simulink model "ARFWr_Sim"  (R2025a)
settings: Solver=ode4  StartTime=0.0  StopTime=simLapStop  FixedStep=2e-4  RelTol=1e-3
PreLoadFcn:
  | % T2.3 ROLLING-START SEAM.
  | %
  | % Plant.slx's model workspace owns plantVx0 (T2.2 report section 4: "a seam,
  | % not a defect"), which drives BOTH the body's xbdot_o and all four tyre blocks'
  | % omegao -- so a rolling start can never be issued with stationary wheels.
  | % Its stored default is 0. This callback pushes the ACTIVE speed target at the
  | % start line into it, so the rolling start matches whatever drvVScale /
  | % drvUsePlan the driver is running with. Plant.slx is NOT this task's file, so
  | % it is not edited: the value is pushed into the loaded model workspace and
  | % Plant's dirty flag is restored, leaving the .slx on disk untouched.
  | %
  | % The vehicle's start POSE needs no push at all -- the reference path in
  | % DriverPath's model workspace was rigidly transformed at build time so that its
  | % first point is the origin with heading 0, which is exactly Plant's stored
  | % Xe_o = eul_o = [0 0 0].
  | %
  | % WHY PreLoadFcn AND NOT InitFcn: a referenced model's workspace is READ-ONLY
  | % once simulation starts. Doing this from InitFcn fails with
  | % Simulink:Libraries:WSLockViolation, "Attempt to modify a read-only model
  | % workspace" -- measured in T2.3. PreLoadFcn runs at load time, outside the lock.
  | %
  | % CONSEQUENCE, and the one thing to know before changing the speed target by
  | % hand: this fires ONCE, when ARFWr_Sim is loaded. If you edit drvVScale or
  | % drvUsePlan in DriverPath's model workspace afterwards and press Run, plantVx0
  | % is STALE and the car starts at the previous speed. Re-run this callback:
  | %     eval(get_param('ARFWr_Sim','PreLoadFcn'))
  | % Scripted runs should instead override it on the SimulationInput, which is
  | % immune to the ordering:
  | %     si = si.setVariable('plantVx0', v0, 'Workspace', 'Plant')
  | load_system('DriverPath');
  | load_system('Plant');
  | mwD = get_param('DriverPath','ModelWorkspace');
  | if mwD.getVariable('drvUsePlan') > 0.5
  |     vProf = mwD.getVariable('drvRefVplan');
  | else
  |     vProf = mwD.getVariable('drvRefVraw');
  | end
  | v0 = mwD.getVariable('drvVScale')*vProf(1);
  | mwP = get_param('Plant','ModelWorkspace');
  | dirty0 = get_param('Plant','Dirty');
  | if ~isequal(mwP.getVariable('plantVx0'), v0)
  |     mwP.assignin('plantVx0', v0);
  |     set_param('Plant','Dirty', dirty0);
  | end
InitFcn:
  | % LIVE INSTRUMENTS -- the DISPLAY-ONLY indicated-gear rule.
  | % indicatedGearParams is the SINGLE owner of ratios/omPk/omCap/nHold, shared
  | % with simulink/viz/indicatedGear.m (the burned-in HUD digit), so the live
  | % Dashboard digit and the recorded video digit cannot drift apart. The plant
  | % runs ONE fixed ratio and never shifts -- see that function's header.
  | hudGear = indicatedGearParams(pt);
model workspace (MAT data in the model file):
  simLapStop = 183
undefined symbols (not defined in the file): Sim3dSensor, vp
libraries: sim3dlib x5, sim3dautolib x1
Description:
  | ARFWr_Sim -- top closed-loop harness (T2.3). NEVER code-generated.
  | 
  | DriverPath -> Plant -> Sensors -> AeroECU -> Plant (wings + TV).
  | Rates: Plant 1 kHz ode4, AeroECU 100 Hz discrete (ecuTs), driver continuous on
  | the parent's 1 ms step.
  | 
  | VARIANTS (both LABEL mode, so the active choice is stored in this .slx and no
  | base-workspace variant control variables are needed):
  |   Scenario Source {ClosedLoop | Replay}  -- ClosedLoop active.
  |   Visualization   {Off | Dashboard | Unreal3D} -- Off active.
  | 
  | SIMULATION PACING is ON at 1x in the saved model, which is what a demo run
  | wants. Every measurement run in T2.3 was made UNPACED, by overriding
  | EnablePacing on a Simulink.SimulationInput -- pacing would make a wall-clock
  | ratio measurement meaningless.
  | 
  | ROLLING START: see this model's InitFcn callback.
  | 
  | STATUS OF THE MODELLING LAYERS (was "PLACEHOLDERS STILL LIVE" until T4.2):
  |   tyres  LIVE  -- per-axle Pacejka MF5.2 (T3.2), gate 1 passes at round-off.
  |   aero   LIVE  -- instantaneous ride-height map + both wing layers (T3.4),
  |                   gate 2 passes; the plant block matches aeroLiveEval to 1e-12.
  |   ECU    LIVE  -- reactive dual-wing law (gate 5, 96/97 % law fidelity) plus,
  |                   since T4.2, the front-axle TV allocator on SensorBus.kappaRef
  |                   and .TqAxle. tv.enable in simulink/params/tvParams.m switches
  |                   TV off at build time.
  |   driver APPROXIMATE -- a forward-time Stanley + traction-pedal-map driver, NOT
  |                   an optimal-control solution. It completes a clean BCN lap in
  |                   138.3 s against the offline solve's 102.674 s (gate 6,
  |                   simulink/validation/validateClosedLoop.m, which prints the
  |                   full wing-schedule and grip-utilisation evidence). Quote the
  |                   gate's own numbers, never an extrapolated partial lap.
settings Model: DataDictionary=ARFWr_RT.sldd  Creator=ASUS  LastModifiedBy=ASUS
settings DataIOCC: SignalLoggingName=simLog
settings DebuggingCC: AlgebraicLoopMsg=error  UnconnectedInputMsg=error  UnconnectedOutputMsg=error  UnconnectedLineMsg=error

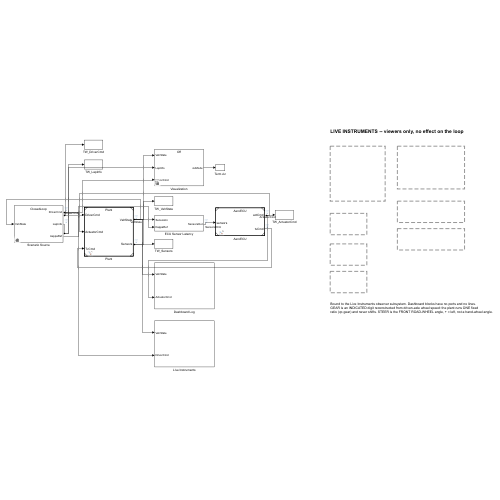
[thumbnail: Simulink's stored preview of the top-level diagram]
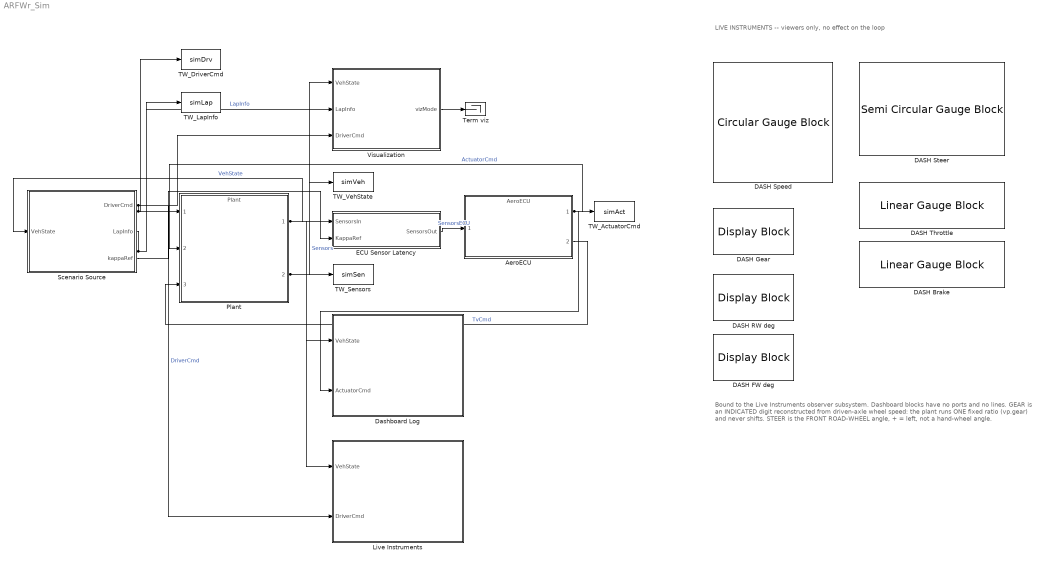
== system ARFWr_Sim ==
  note: LIVE INSTRUMENTS -- viewers only, no effect on the loop
  note: Bound to the Live Instruments observer subsystem. Dashboard blocks have no ports and no lines.
      | GEAR is an INDICATED digit reconstructed from driven-axle wheel speed: the plant runs ONE fixed
      | ratio (vp.gear) and never shifts. STEER is the FRONT ROAD-WHEEL angle, + = left, not a hand-wheel angle.
  AeroECU : ModelReference  Description=AeroECU (T1.1-T1.5), 100 Hz discrete (ecuTs = 0.01). Sensors in, ActuatorCmdBus + TvCmdBus out. NOT tuned or touched by T2.3.  ModelNameDialog=AeroECU  SimulationMode=Normal  ModelReferenceVersion=1.7
  DASH Brake : LinearGaugeBlock  Description="BRAKE  %"  LabelPosition=Bottom  FontColor=[0.0, 0.0, 0.0]
  DASH FW deg : DisplayBlock  Description="FRONT FLAP alphaFW_pos  [deg]"  LabelPosition=Bottom  Transparency=1  GridColor=[0.502, 0.502, 0.502]
  DASH Gear : DisplayBlock  Description=GEAR (indicated) -- plant runs one ratio, never shifts  LabelPosition=Bottom  Transparency=1  GridColor=[0.502, 0.502, 0.502]
  DASH RW deg : DisplayBlock  Description="REAR WING alphaRW_pos  [deg]"  LabelPosition=Bottom  Transparency=1  GridColor=[0.502, 0.502, 0.502]
  DASH Speed : CircularGaugeBlock  Description="SPEED  km/h"  LabelPosition=Bottom  ScaleMax=360  FontColor=[0.0, 0.0, 0.0]
  DASH Steer : SemiCircularGaugeBlock  Description="STEER road-wheel, + = left  [deg]"  LabelPosition=Bottom  ScaleMin=-15  ScaleMax=15  FontColor=[0.0, 0.0, 0.0]
  DASH Throttle : LinearGaugeBlock  Description="THROTTLE  %"  LabelPosition=Bottom  FontColor=[0.0, 0.0, 0.0]
  Dashboard Log : Subsystem  Description=|
      | T5.2 dashboard logging tap (simulink/viz/dashboardApp.m's SIGNAL-NAME CONTRACT).
      | Pure observer: two Inports branch the existing VehState and ActuatorCmd lines,
      | nothing is fed back into the loop and every output ends in a Terminator, so the
      | closed loop is bit-identical with this subsystem present or deleted.
      | 
      | Every logged port uses DataLoggingNameMode = Custom, so the logsout element name
      | is fixed by this block and cannot drift with a line label:
      |   vehState.x vehState.y           -- flat elements whose NAME carries the dot
      |   vx                              -- plant truth off VehStateBus (NOT the
      |                                      latency-delayed SensorBus copy)
      | alphaRW_pos / alphaFW_pos are NOT tapped here: Plant.slx already logs both
      | under exactly those names, and two same-named Dataset elements break
      | getElement(name) lookup (it returns a Dataset of the matches, not an
      | element). The tap copy was measured bit-identical to Plant's.
      |   stationRW stationFW sOn         -- ActuatorCmdBus; the stations are the
      |                                      1-BASED INDEX the contract asks for, not degrees
      |   aeroClF aeroClR aeroCd          -- optional north-star downforce/drag panel
  ECU Sensor Latency : Subsystem  Description=|
      | ONE-SAMPLE (1 ms) SENSOR LATENCY on the Plant -> AeroECU path. This is the
      | ALGEBRAIC-LOOP BREAK for the ECU half of the closed loop -- the driver half is
      | broken separately, inside DriverPath (see its Sensor delay block).
      | 
      | MEASURED, not assumed. Wiring Plant.Sensors straight into AeroECU.sensors gives:
      |   Simulink:Engine:BlockWithStatesModifiedInOutputUpdateInAlgLoop
      |     "ARFWr_Sim/Plant or the model referenced by it contains a block that updates
      |      persistent or state variables while computing outputs and is not supported
      |      in an algebraic loop"
      |   Simulink:Engine:BlkWithPortInLoop  input ports (1,2,3,4) of ARFWr_Sim/AeroECU
      |   Simulink:Engine:BlkWithPortInLoop  input ports (4..9) of ARFWr_Sim/Plant
      | i.e. Sensors -> ECU -> ActuatorCmd/TvCmd -> Plant -> Sensors. The offending
      | stateful block is the VDB Combined Slip Wheel 2DOF (its Wheel Module clutch
      | updates state while computing outputs), which is the same block T2.2 already had
      | to break with a Memory on the Omega feedback -- see Plant/Omega Memory.
      | 
      | PHYSICALLY HONEST, not a workaround: the ECU is a 100 Hz sampled controller
      | reading sensors over a bus. One 1 ms sample of acquisition latency is an order
      | of magnitude LESS than the 10 ms the controller already waits between its own
      | steps, so it changes nothing the ECU can observe.
      | 
      | Mux/Demux around the Memory because SensorBus is a VIRTUAL bus and Memory does
      | not accept one. Channel order is the Bus Selector's: vx, r, Tbrake, TbMax.
  Live Instruments : Subsystem  Description=|
      | LIVE INSTRUMENTS -- pure observer for the root Dashboard blocks.
      | 
      | Two Inports BRANCH the existing top-level VehState (Plant/1) and DriverCmd
      | (Scenario Source/1) lines. Nothing is fed back into the loop and every signal
      | ends in a Terminator, so the closed loop is bit-identical with this subsystem
      | present or deleted -- the same contract as the Dashboard Log tap next door.
      | 
      | Display units, so the gauges read what a driver would read:
      |   Speed kmh    = vx * 3.6            [km/h]
      |   Steer deg    = steer * 180/pi      [deg, FRONT ROAD-WHEEL angle, + = LEFT --
      |                                       NOT a hand-wheel angle; peak ~11 deg]
      |   Throttle pct = accel * 100         [%, POST traction ceiling]
      |   Brake pct    = brake * 100         [%, POST traction ceiling]
      |   alphaRW_pos / alphaFW_pos pass through unscaled -- already degrees.
      | 
      | GEAR OBSERVER -- DISPLAY ONLY, and the caveat travels with the number.
      | Plant.slx models ONE fixed effective ratio (vp.gear) and NEVER SHIFTS; the
      | supplier 8-speed table pt.gearbox is read by nothing in the plant or the
      | solver. This block reconstructs a legibility digit from driven-axle wheel
      | speed at 0.05 s, the same rule and the same parameters as
      | simulink/viz/indicatedGear.m (single owner: indicatedGearParams). No shift
      | event, torque interruption, ratio step or inertia change exists anywhere in
      | the simulation, and no reported result depends on this digit. It must never
      | appear in a lap-time, shift-strategy or powertrain statement.
      | 
      | Every gear parameter arrives as a Constant whose Value is a hudGear field, so
      | there is no numeric literal in the gear path. hudGear is built by the model
      | InitFcn as indicatedGearParams(pt).
  Plant : ModelReference  Description=|  ModelNameDialog=Plant  SimulationMode=Normal  ModelReferenceVersion=1.14
      | Plant.slx (T2.2), 1 kHz ode4. In: DriverCmd, ActuatorCmd, TvCmd. Out: VehState
      | (full state, ISO 8855), Sensors (the four channels the ECU consumes).
      | Not touched by T2.3 -- see this model's InitFcn for the one runtime value
      | (plantVx0) that is pushed into its model workspace and immediately un-dirtied.
  Scenario Source : Subsystem  Description=|  Variant=on  VariantControlMode=label  LabelModeActiveChoice=ClosedLoop
      | ScenarioSource variant (design spec decision 2, "closed loop + replay mode").
      | Label mode; active choice ClosedLoop. Both choices take VehStateBus in and
      | produce DriverCmdBus + a 12-element LapInfo vector out.
  TW_ActuatorCmd : ToWorkspace  VariableName=simAct  SaveFormat=Structure With Time  SampleTime=-1
  TW_DriverCmd : ToWorkspace  VariableName=simDrv  SaveFormat=Structure With Time  SampleTime=-1
  TW_LapInfo : ToWorkspace  VariableName=simLap  SaveFormat=Structure With Time  SampleTime=-1
  TW_Sensors : ToWorkspace  VariableName=simSen  SaveFormat=Structure With Time  SampleTime=-1
  TW_VehState : ToWorkspace  VariableName=simVeh  SaveFormat=Structure With Time  SampleTime=-1
  Term viz : Terminator
  Visualization : Subsystem  Description=|  Variant=on  VariantControlMode=label  LabelModeActiveChoice=Off
      | Visualization variant (design spec decision 10: "Viz outside RT boundary").
      | Label mode; active choice Off. All three choices take VehState + LapInfo and
      | return a scalar vizMode indicator (0 Off, 1 Dashboard, 2 Unreal3D) so the
      | active choice is observable in a log without opening the model.
      | 
      | All three choices are implemented: Off is a pure pass-through terminator
      | (T5.0), Dashboard is the logged-lap replay dashboard (T5.1/T5.2), Unreal3D
      | is the live sim3d scene (T5.3). None is a stub.
  wires:
  ECU Sensor Latency/1(SensorsOut) -> AeroECU/1  "SensorsECU"
  Scenario Source/1(DriverCmd) -> Plant/1, TW_DriverCmd/1, Live Instruments/2(DriverCmd), Visualization/3(DriverCmd)  "DriverCmd"
  Scenario Source/2(LapInfo) -> Visualization/2(LapInfo), TW_LapInfo/1  "LapInfo"
  Plant/1 -> Scenario Source/1(VehState), Visualization/1(VehState), TW_VehState/1, Dashboard Log/1(VehState), Live Instruments/1(VehState)  "VehState"
  AeroECU/1 -> Plant/2, TW_ActuatorCmd/1, Dashboard Log/2(ActuatorCmd)  "ActuatorCmd"
  Plant/2 -> TW_Sensors/1, ECU Sensor Latency/1(SensorsIn)  "Sensors"
  AeroECU/2 -> Plant/3  "TvCmd"
  Visualization/1(vizMode) -> Term viz/1
  Scenario Source/3(kappaRef) -> ECU Sensor Latency/2(KappaRef)

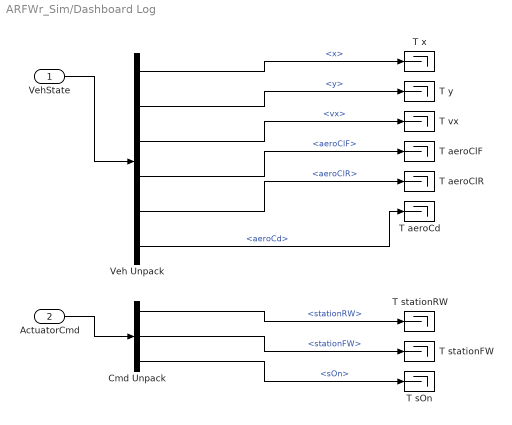
== system ARFWr_Sim/Dashboard Log ==
  VehState : Inport
  ActuatorCmd : Inport  Port=2
  Cmd Unpack : BusSelector  OutputSignals=stationRW,stationFW,sOn
  T aeroCd : Terminator
  T aeroClF : Terminator
  T aeroClR : Terminator
  T sOn : Terminator
  T stationFW : Terminator
  T stationRW : Terminator
  T vx : Terminator
  T x : Terminator
  T y : Terminator
  Veh Unpack : BusSelector  OutputSignals=x,y,vx,aeroClF,aeroClR,aeroCd
  wires:
  VehState/1 -> Veh Unpack/1
  ActuatorCmd/1 -> Cmd Unpack/1
  Veh Unpack/1 -> T x/1  "<x>"
  Veh Unpack/2 -> T y/1  "<y>"
  Veh Unpack/3 -> T vx/1  "<vx>"
  Veh Unpack/4 -> T aeroClF/1  "<aeroClF>"
  Veh Unpack/5 -> T aeroClR/1  "<aeroClR>"
  Veh Unpack/6 -> T aeroCd/1  "<aeroCd>"
  Cmd Unpack/1 -> T stationRW/1  "<stationRW>"
  Cmd Unpack/2 -> T stationFW/1  "<stationFW>"
  Cmd Unpack/3 -> T sOn/1  "<sOn>"

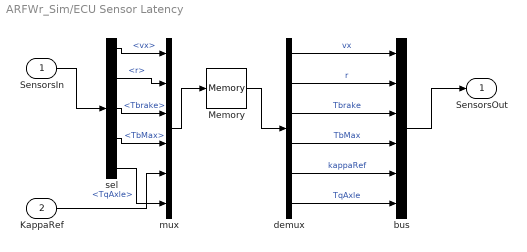
== system ARFWr_Sim/ECU Sensor Latency ==
  SensorsIn : Inport  OutDataTypeStr=Bus: SensorBus
  KappaRef : Inport  Description=Path curvature at the preview point, ISO [1/m], straight from the Scenario Source. It is muxed in as SensorBus element 5 INSTEAD of the element the Plant publishes (which is a hard 0 -- the plant has no path knowledge). Delayed by the same one 1 ms Memory sample as the plant channels so the ECU sees one consistent sensor snapshot.  Port=2
  Memory : Memory  Description=|  InitialCondition=[0; 0; 0; vp.Tbrake_max; 0; 0]
      | Initial condition [0; 0; 0; vp.Tbrake_max].
      | 
      | The fourth entry MUST be vp.Tbrake_max and MUST NOT be left at 0. SensorBus.TbMax
      | is the POSITIVE brake-torque magnitude cap, and the reactive law's brake trigger
      | (Functions/rwVelocityTarget.m's brakeSwitch, ported into AeroECU) uses an onset
      | width of w1frac*TbMax -- so a zero TbMax on the very first step divides by zero
      | inside the tanh argument. This is the same contract Plant's Vehicle State Bus
      | subsystem documents ("TbMax > 0 ALWAYS").
      | 
      | vx = r = Tbrake = 0 for one 1 ms step is harmless: kap2 = r^2/(vx^2+1) is 0
      | there, and Tbrake = 0 simply means "not braking" on step one.
  bus : BusCreator  Inputs=6  OutDataTypeStr=Bus: SensorBus
  demux : Demux  Outputs=6
  mux : Mux  Inputs=6
  sel : BusSelector  OutputSignals=vx,r,Tbrake,TbMax,TqAxle
  SensorsOut : Outport  OutDataTypeStr=Bus: SensorBus
  wires:
  SensorsIn/1 -> sel/1
  sel/1 -> mux/1  "<vx>"
  demux/1 -> bus/1  "vx"
  sel/2 -> mux/2  "<r>"
  demux/2 -> bus/2  "r"
  sel/3 -> mux/3  "<Tbrake>"
  demux/3 -> bus/3  "Tbrake"
  sel/4 -> mux/4  "<TbMax>"
  demux/4 -> bus/4  "TbMax"
  mux/1 -> Memory/1
  Memory/1 -> demux/1
  bus/1 -> SensorsOut/1
  sel/5 -> mux/6  "<TqAxle>"
  KappaRef/1 -> mux/5
  demux/5 -> bus/5  "kappaRef"
  demux/6 -> bus/6  "TqAxle"

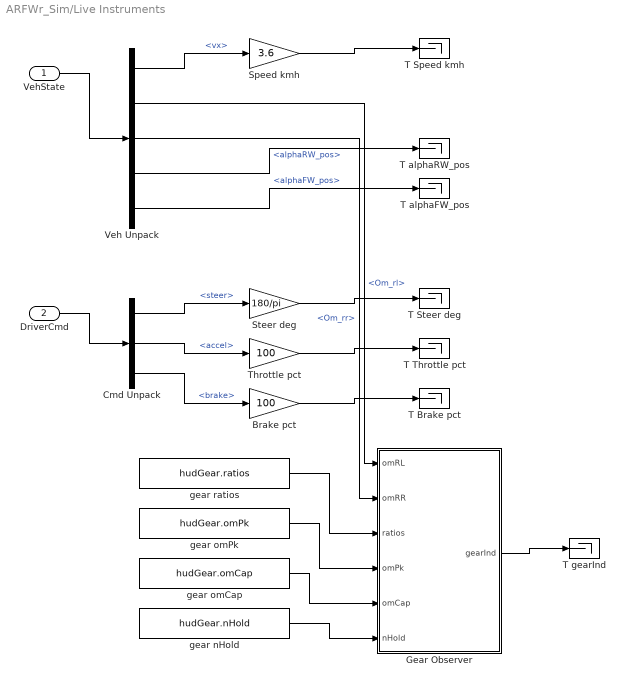
== system ARFWr_Sim/Live Instruments ==
  VehState : Inport
  DriverCmd : Inport  Port=2
  Brake pct : Gain  Description=DriverCmdBus.brake [0..1, POST traction ceiling] -> percent. Sampled at 0.05 s; display only.  Gain=100  SampleTime=0.05
  Cmd Unpack : BusSelector  OutputSignals=steer,accel,brake
  Gear Observer : MATLAB Function  Description=|  TreatAsAtomicUnit=on
      | DISPLAY-ONLY indicated gear, live. Reproduces simulink/viz/indicatedGear.m's
      | rule sample by sample: of the eight candidate crank speeds omWheel*ratios,
      | take the one nearest omPk among those at or under omCap (all over cap -> top
      | gear), then hold the digit until a new candidate has persisted nHold samples.
      | The plant runs ONE fixed ratio and never shifts -- this digit is a legibility
      | aid, never a shift model, and no reported result depends on it.
  Speed kmh : Gain  Description=vx [m/s] -> km/h for the speed Gauge. Sampled at 0.05 s; display only.  Gain=3.6  SampleTime=0.05
  Steer deg : Gain  Description=DriverCmdBus.steer [rad] -> deg. FRONT ROAD-WHEEL angle, + = LEFT, NOT a hand-wheel angle. Sampled at 0.05 s; display only.  Gain=180/pi  SampleTime=0.05
  T Brake pct : Terminator
  T Speed kmh : Terminator
  T Steer deg : Terminator
  T Throttle pct : Terminator
  T alphaFW_pos : Terminator
  T alphaRW_pos : Terminator
  T gearInd : Terminator
  Throttle pct : Gain  Description=DriverCmdBus.accel [0..1, POST traction ceiling] -> percent. Sampled at 0.05 s; display only.  Gain=100  SampleTime=0.05
  Veh Unpack : BusSelector  OutputSignals=vx,Om_rl,Om_rr,alphaRW_pos,alphaFW_pos
  gear nHold : Constant  Description=Dwell-filter length in samples, round(Dwell/Dt). From indicatedGearParams(pt).  Value=hudGear.nHold
  gear omCap : Constant  Description=Candidate mask: min(ICE redline, e-motor ceiling referred to the crank) [rad/s]. From indicatedGearParams(pt).  Value=hudGear.omCap
  gear omPk : Constant  Description=Crank speed at the ICE map's OWN peak power [rad/s]. From indicatedGearParams(pt).  Value=hudGear.omPk
  gear ratios : Constant  Description=Overall ratio wheel -> crank, pt.FD * pt.gearbox. From indicatedGearParams(pt) via the model InitFcn -- no literal here.  Value=hudGear.ratios
  wires:
  VehState/1 -> Veh Unpack/1
  DriverCmd/1 -> Cmd Unpack/1
  Veh Unpack/1 -> Speed kmh/1  "<vx>"
  Speed kmh/1 -> T Speed kmh/1
  Cmd Unpack/1 -> Steer deg/1  "<steer>"
  Steer deg/1 -> T Steer deg/1
  Cmd Unpack/2 -> Throttle pct/1  "<accel>"
  Throttle pct/1 -> T Throttle pct/1
  Cmd Unpack/3 -> Brake pct/1  "<brake>"
  Brake pct/1 -> T Brake pct/1
  Veh Unpack/4 -> T alphaRW_pos/1  "<alphaRW_pos>"
  Veh Unpack/5 -> T alphaFW_pos/1  "<alphaFW_pos>"
  Veh Unpack/2 -> Gear Observer/1(omRL)  "<Om_rl>"
  Veh Unpack/3 -> Gear Observer/2(omRR)  "<Om_rr>"
  gear ratios/1 -> Gear Observer/3(ratios)
  gear omPk/1 -> Gear Observer/4(omPk)
  gear omCap/1 -> Gear Observer/5(omCap)
  gear nHold/1 -> Gear Observer/6(nHold)
  Gear Observer/1(gearInd) -> T gearInd/1

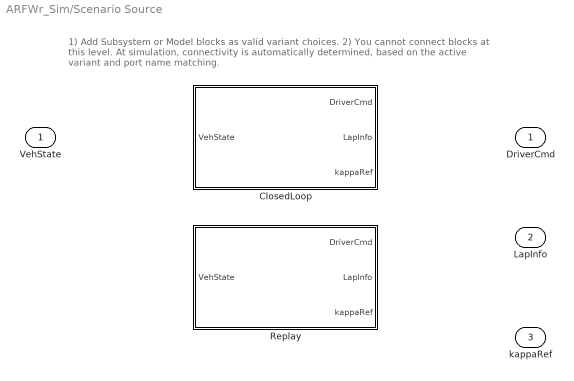
== system ARFWr_Sim/Scenario Source ==
  note: 1) Add Subsystem or Model blocks as valid variant choices.
      | 2) You cannot connect blocks at this level. At simulation, connectivity is automatically
      | determined, based on the active variant and port name matching.
  VehState : Inport  OutDataTypeStr=Bus: VehStateBus
  ClosedLoop : Subsystem  Description=|  VariantControl=ClosedLoop
      | ClosedLoop: the DriverPath model reference drives the vehicle round the solved
      | ARFWr racing line. See DriverPath.slx's own description for the reference
      | construction, the vehicle-frame preview trick and the traction pedal map.
  Replay : Subsystem  Description=|  VariantControl=Replay
      | Replay: STUB (T2.3 scope -- the brief allows a stub referencing the working
      | replay model). The real replay path already exists as a standalone model,
      | simulink/models/ARFWr_Replay.slx (T1.6, gate 5 PASS: law fidelity RW 96.09 % /
      | FW 97.49 % station agreement), driven by simulink/tools/buildReplayInput.m,
      | which reads recorded vx / r / Tbrake / TbMax straight out of
      | solutions/report/BCN/raw/run_BCN_ARFWr_ATD_data.mat and plays them into the ECU
      | open-loop. Folding that pattern in here means driving THIS model's AeroECU from
      | the same recorded SensorBus instead of from the Plant -- i.e. the replay choice
      | has to override the SENSOR path, not the driver path, so it is a slightly
      | larger change than swapping this subsystem. It is left as a stub deliberately.
      | 
      | What the stub does: terminates VehState, emits a zero DriverCmd (steer 0,
      | accel 0, brake 0) and a zero LapInfo of the same 12x1 shape the ClosedLoop
      | choice produces. Selecting it leaves the car coasting from its rolling start.
  DriverCmd : Outport  OutDataTypeStr=Bus: DriverCmdBus
  LapInfo : Outport  Port=2
  kappaRef : Outport  Description=Reference-path curvature [1/m] at the driver preview point, ISO 8855 (+ = LEFT). Feeds SensorBus.kappaRef via ECU Sensor Latency, for the AeroECU TV allocator only. ClosedLoop sources it from DriverPath; Replay emits 0 (no path).  Port=3

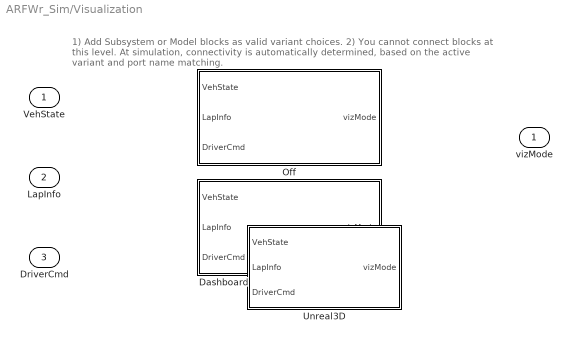
== system ARFWr_Sim/Visualization ==
  note: 1) Add Subsystem or Model blocks as valid variant choices.
      | 2) You cannot connect blocks at this level. At simulation, connectivity is automatically
      | determined, based on the active variant and port name matching.
  VehState : Inport  OutDataTypeStr=Bus: VehStateBus
  LapInfo : Inport  Port=2
  DriverCmd : Inport  Port=3  OutDataTypeStr=Bus: DriverCmdBus
  Dashboard : Subsystem  Description=|  VariantControl=Dashboard
      | Dashboard -- STUB, owned by T5.1. Intended contents: the 2D dashboard of
      | simulink/viz/dashboardApp.m at ~50 ms (design spec: "dashboard 50 ms"),
      | plus a track-ribbon XY trace driven off VehState.x/y and LapInfo(1) sLap.
      | Terminators mark the seam, exactly as the Plant's T3.4 aero seam does.
  Off : Subsystem  Description=Off (default). Terminates both inputs. Zero cost, and the only choice that belongs in a wall-clock/RT measurement.  VariantControl=Off
  Unreal3D : Subsystem  Description=|  VariantControl=Unreal3D
      | Unreal (sim3d) 3D view of the live closed loop, drawn on the SAME car as
      | the offline route: simulink/viz/zenvoCarActors.m with assetManifest('Zenvo'),
      | on the Barcelona ribbon from buildTrackRibbon. One Simulation 3D Actor
      | block ("Car") builds the whole hierarchy in its init script and drives every
      | moving part by actor NAME -- body pose, four steering/spinning wheels, the
      | transplanted rear wing, the two-strip front flap's shared hinge, and the
      | three station bands.
      | Pure observer -- no signal is fed back, so the closed loop is unchanged
      | whichever choice is active.
      | 
      | The 3D WINDOW rides the car: the init script re-parents World.Viewports.Main
      | onto the car's own CamRig (front-3/4). That closes the rad/deg camera
      | limitation for the window. The in-model capture camera (RecCam) still needs
      | a vehTag-able mount, so it rides "CamCarrier" -- a Simulation 3D Vehicle
      | scaled to 0.001 and fed the pose in RADIANS, with its mount offset
      | pre-multiplied by 1000 to survive that scale. RecCam is a CHASE view for
      | documentation frames only, terminated and unlogged by default.
      | 
      | Wing and wheel GEOMETRY is the asset's; the ANGLES are the model's own
      | numbers. Wheel spin is presented with a cosmetic per-frame cap by default
      | (spinModeApparent = 1) and is never a measurable wheel speed. Certified
      | full-lap footage still comes from simulink/viz/unrealPlayback.m.
  vizMode : Outport

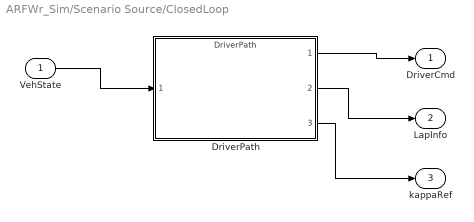
== system ARFWr_Sim/Scenario Source/ClosedLoop ==
  VehState : Inport  OutDataTypeStr=Bus: VehStateBus
  DriverPath : ModelReference  ModelNameDialog=DriverPath  SimulationMode=Normal  ModelReferenceVersion=1.18
  DriverCmd : Outport  OutDataTypeStr=Bus: DriverCmdBus
  LapInfo : Outport  Port=2
  kappaRef : Outport  Port=3
  wires:
  VehState/1 -> DriverPath/1
  DriverPath/1 -> DriverCmd/1
  DriverPath/2 -> LapInfo/1
  DriverPath/3 -> kappaRef/1

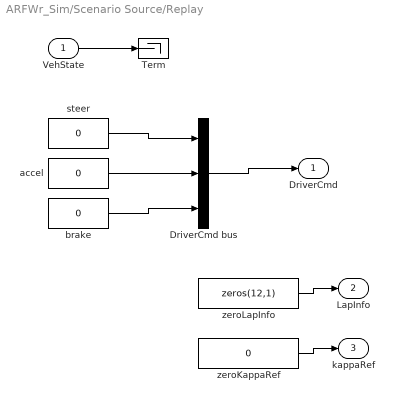
== system ARFWr_Sim/Scenario Source/Replay ==
  VehState : Inport  OutDataTypeStr=Bus: VehStateBus
  DriverCmd bus : BusCreator  Inputs=3  OutDataTypeStr=Bus: DriverCmdBus
  Term : Terminator
  accel : Constant  Description=STUB, see the steer constant.  Value=0
  brake : Constant  Description=STUB, see the steer constant.  Value=0
  steer : Constant  Description=STUB. Replay drives the ECU open-loop from recorded vx/r/Tbrake; the vehicle is not driven at all, so the driver command is zero. See simulink/models/ARFWr_Replay.slx (T1.6) for the working replay model and simulink/tools/buildReplayInput.m for the signal source.  Value=0
  zeroKappaRef : Constant  Description=STUB, matching the ClosedLoop choice's third output. The replay stub does not drive the vehicle and has no path reference, so the TV allocator's yaw-rate target is 0 and the allocator only damps yaw. Same reasoning as Plant's own sb.kappaRef = 0.  Value=0
  zeroLapInfo : Constant  Description=STUB. LapInfo shape must match the ClosedLoop choice (12x1); see DriverPath's LapInfo outport description for the index table.  Value=zeros(12,1)
  DriverCmd : Outport  OutDataTypeStr=Bus: DriverCmdBus
  LapInfo : Outport  Port=2
  kappaRef : Outport  Port=3
  wires:
  VehState/1 -> Term/1
  steer/1 -> DriverCmd bus/1
  accel/1 -> DriverCmd bus/2
  brake/1 -> DriverCmd bus/3
  DriverCmd bus/1 -> DriverCmd/1
  zeroLapInfo/1 -> LapInfo/1
  zeroKappaRef/1 -> kappaRef/1

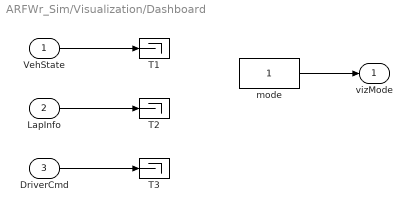
== system ARFWr_Sim/Visualization/Dashboard ==
  VehState : Inport  OutDataTypeStr=Bus: VehStateBus
  LapInfo : Inport  Port=2
  DriverCmd : Inport  Port=3  OutDataTypeStr=Bus: DriverCmdBus
  T1 : Terminator
  T2 : Terminator
  T3 : Terminator
  mode : Constant  Description=Active-choice indicator: 1 = Dashboard. Value 1 is the Constant-block factory default; the SLX writer strips default-valued parameters, so it cannot be stored explicitly in the .slx -- effective value verified 1. Siblings DO store theirs (Off = 0, Unreal3D = 2), so only this one relies on the default.
  vizMode : Outport
  wires:
  VehState/1 -> T1/1
  LapInfo/1 -> T2/1
  mode/1 -> vizMode/1
  DriverCmd/1 -> T3/1

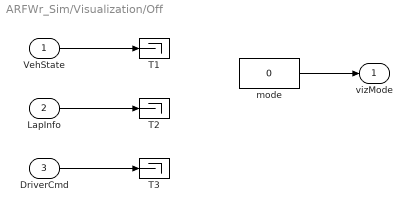
== system ARFWr_Sim/Visualization/Off ==
  VehState : Inport  OutDataTypeStr=Bus: VehStateBus
  LapInfo : Inport  Port=2
  DriverCmd : Inport  Port=3  OutDataTypeStr=Bus: DriverCmdBus
  T1 : Terminator
  T2 : Terminator
  T3 : Terminator
  mode : Constant  Description=Active-choice indicator: 0 = Off.  Value=0
  vizMode : Outport
  wires:
  VehState/1 -> T1/1
  LapInfo/1 -> T2/1
  mode/1 -> vizMode/1
  DriverCmd/1 -> T3/1

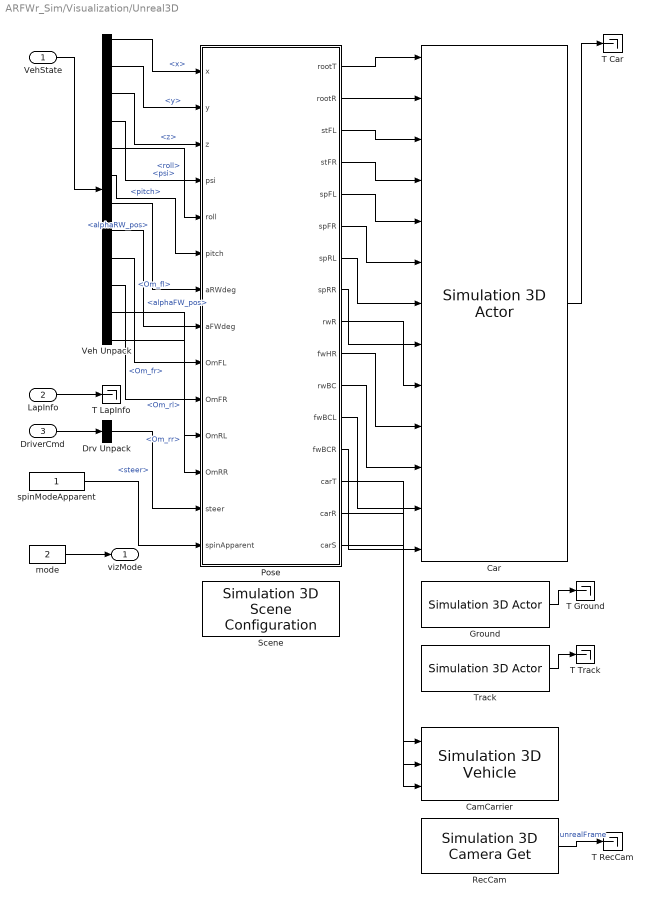
== system ARFWr_Sim/Visualization/Unreal3D ==
  VehState : Inport
  LapInfo : Inport  Port=2
  DriverCmd : Inport  Port=3
  CamCarrier : sim3dautolib/Simulation 3D Vehicle  Priority=-1  PassVehMesh=Muscle car  MeshPath=/MathWorksAutomotiveContent/Vehicles/Muscle/Meshes/SK_MuscleCar.SK_MuscleCar  VehColor=Red  ActorName=SimulinkVehicle1  VehLightsControl=off  HeadlightColor=[ 1, 1, 1 ]  HighBeamIntensity=100000  LowBeamIntensity=60000  HighBeamConeAngle=1.22  LowBeamConeAngle=1.22  LeftHeadlightOrientation=[ 0, 0 ]  RightHeadlightOrientation=[ 0, 0 ]  BrakelightIntensity=500  ReverselightIntensity=500  SignallightIntensity=500  SignallightPeriod=1  SignalPulseWidth=50  Translation=zeros( 5, 3 )  Rotation=zeros( 5, 3 )  Scale=ones( 5, 3 )  SampleTime=0.05  ActorType=SimulinkVehicle  ID=1  aMode=2  ActorTag=SimulinkVehicle1
      settings: LibrarySourceBlock=vehdynlibsim3d/Simulation 3D Vehicle
  Car : sim3dlib/Simulation 3D Actor  Description=|  Priority=1  ActorName=CarHost  ParentName=Scene Origin  Operation=Create at setup  InitScriptText=|  SampleTime=0.05  Translation=[0 0 0]  Rotation=[0 0 0]  Scale=[1 1 1]  InputsText=|  aMode=aMode  ActorTag=CarHost  ActorType=Sim3dActor  ID=3
      Description=|
      | The whole car: simulink/viz/zenvoCarActors.m + assetManifest('Zenvo').
      | InputsText addresses each moving part by the actor names that builder
      | freezes. The three .Color lines (11-13) recolour the rear wing's station
      | band and the two front-flap bands from dashboardApp's palette; the
      | Simulation 3D Actor block accepts .Color as an input the same way it
      | accepts .Rotation (measured, not assumed). The colour goes on the BANDS
      | and never on a surface: every part of this asset is a texture on a white
      | material, so painting a surface would paint over the car's own skin.
      | The init script re-parents the car root under THIS block's actor --
      | InputsText only reaches descendants of it, and a top-level root renders
      | at the world origin and never moves. It also re-parents
      | World.Viewports.Main onto the car's own CamRig, which is what makes the
      | 3D WINDOW ride the car.
      InitScriptText=|
      | % A 1 cm marker so the BLOCK's own actor certainly spawns: it is the
      | % parent the whole car hangs off, and it never moves from the world origin.
      | createShape(Actor, 'box', [0.01 0.01 0.01]);
      | Actor.CoordinateSystem = 'ISO8855';
      | % The imported car, its wheels and every actuated aero surface, under ONE
      | % ISO8855 root. Single owner: simulink/viz/zenvoCarActors.m.
      | vpB = evalin('base', 'vp');
      | HC  = zenvoCarActors(World, vpB, assetManifest('Zenvo'));
      | % RE-PARENT, and it is NOT cosmetic. zenvoCarActors adds its root at the
      | % top of the world; this block's InputsText only reaches actors that are
      | % DESCENDANTS of the block's own actor. Measured 2026-09-17 with the same
      | % camera on both sides of this one line: without it the car renders at the
      | % world origin and never moves (Root.Translation still READS BACK as the
      | % commanded value through OutputsText, so the read-back alone does not
      | % catch it -- only a frame does); with it the car follows its input.
      | add(World, HC.root, Actor);
      | % The viewer WINDOW rides the car: the rig is a child of the car root, so
      | % the window follows the body through the whole lap. No vehTag, so no
      | % radians/degrees mismatch (docs/simulink-arfwr-rt.md limitation 9).
      | %
      | % NO try/catch. A window that quietly falls back to a fixed view is a
      | % DEFECT for this variant -- the whole point of it is that the 3D view
      | % rides the car -- and it is a defect nobody watching a render would
      | % report as a failure. So the re-parent is a plain assignment and its
      | % result is read back and asserted.
      | mc = World.Viewports.Main;
      | mc.Parent = HC.camRig;
      | mc.CoordinateSystem = 'ISO8855';
      | mc.Translation = [0 0 0];
      | mc.Rotation    = [0 0 0];
      | mcP  = mc.Parent;
      | mcPN = '<none>';
      | if ~isempty(mcP), mcPN = mcP.Name; end
      | assert(strcmp(mcPN, HC.camRig.Name), 'buildUnreal:mainCamParent', ...
      |     'Unreal3D: viewer camera parent is "%s", expected "%s" -- the 3D window would show a FIXED view while the car drives away.', ...
      |     mcPN, HC.camRig.Name);
      InputsText=|
      | Root.Translation
      | Root.Rotation
      | SteerFL.Rotation
      | SteerFR.Rotation
      | SpinFL.Rotation
      | SpinFR.Rotation
      | SpinRL.Rotation
      | SpinRR.Rotation
      | WingRW.Rotation
      | WingFWHinge.Rotation
      | WingRWBand.Color
      | WingFWBandL.Color
      | WingFWBandR.Color
  Drv Unpack : BusSelector  OutputSignals=steer
  Ground : sim3dlib/Simulation 3D Actor  Priority=1  ActorName=Ground  ParentName=Scene Origin  Operation=Create at setup  InitScriptText=|  SampleTime=0.05  Translation=[422.9169 -88.15729 -0.55]  Rotation=[0 0 0]  Scale=[1 1 1]  aMode=aMode  ActorTag=Ground  ActorType=Sim3dActor  ID=1
      | % Ground slab sized to the ribbon, because the shipped scenes' ground
      | % tile is finite and BCN runs off it (T5.3).
      | % PlantFrame, true: same frame as the Track actor below -- see there.
      | rib = buildTrackRibbon('', 'PlantFrame', true);
      | e  = [rib.lanes.kerbLouter; rib.lanes.kerbRouter];
      | bb = [min(e(:,1)) max(e(:,1)); min(e(:,2)) max(e(:,2))];
      | createShape(Actor, 'box', [diff(bb(1,:))+500, diff(bb(2,:))+500, 1.0]);
      | Actor.CoordinateSystem = 'ISO8855';
      | Actor.Translation = [mean(bb(1,:)), mean(bb(2,:)), -0.55];
      | Actor.Color = [0.30 0.38 0.22];
      | Actor.Metallic = 0; Actor.Specular = 0.02; Actor.Shadows = false;
  Pose : MATLAB Function  TreatAsAtomicUnit=on
  RecCam : sim3dlib/Simulation 3D Camera Get  Description=|  Priority=1  sensorTag=Sim3dSensor�  sensorId=1  sensorName=Sim3dSensor�  vehTagList={'CarHost';'Ground';'Scene Origin';'Sim3dActor1';'Sim3dActor2';'Sim3dActor3';'SimulinkVehicle1';'Track'}  vehTag=SimulinkVehicle1  CoordinateSystem=Default  mountLoc=Origin  offsetFlag=on  tmountOffset=[-12000, 900, 1800]  rmountOffset=[0, 0, 0]  HorizontalResolution=1280  VerticalResolution=720  HorizontalFOV=75  SampleTime=0.05  mountPoint=[-12000 900 1800]  mountOrientation=[0 0 0]  aMode=aMode  ID=1
      | Documentation frames only: terminated and UNLOGGED by default. The lap-
      | time and schedule evidence comes from the gates, never from a render.
      | 
      | Chase mount on "CamCarrier", 12 m back / 0.9 m across / 1.8 m up. Offsets
      | are x1000 because tmountOffset scales with the carrier's 0.001 Scale
      | input, and rmountOffset is zero because the camera already looks along the
      | carrier's +x (that also sidesteps the mask prompt reading "(deg)" while
      | the block consumes RADIANS).
      | 
      | STANDOFF SKEW: the carrier pose and the car root pose are written by the
      | same Pose step, but the engine may draw them one render tick apart, so the
      | apparent standoff moves with speed -- about 3.4 m at 69 m/s. The 12 m
      | mount carries that as headroom; a 9 m mount cropped the car at high speed.
      | This is a framing artefact of the capture camera only. It does not touch
      | the viewer WINDOW, which is parented to the car's own CamRig and moves
      | with it exactly.
  Scene : sim3dlib/Simulation 3D Scene Configuration  Priority=0  ProjectFormat=Default Scenes  SceneDesc=Empty Grass  ProjectName=D:\Software Installs\MATLAB\R2025a\toolbox\shared\sim3d_projects\automotive_project_windows\UE\WindowsNoEditor\VehicleSimulation.exe  ScenePath=/Game/Maps/EmptyGrass4k4k  EnableOpenDRIVE=off  vehTagList={'Custom';'Scene Origin'}  vehTag=Scene Origin  AttachedCameraRelativeTranslation=[0 0 0]  FreeCameraDefaultInitialTranslation=[-6, 0, 2]  AttachedCameraRelativeRotation=[0 0 0]  FreeCameraDefaultInitialRotation=[0, -15, 0]  ViewpointName=Custom  FreeCameraInitialTranslation=[0 0 0]  ViewpointTranslation=[0 0 0]  FreeCameraInitialRotation=[0 0 0]  ViewpointRotation=[0 0 0]  OpVisEn=off  Ts=0.05  EnableWindow=on  EnableRemoteAccess=off  EnableWeather=off  SunAzimuth=90  SunAltitude=40.0  EnableGeospatialSun=off  Latitude=0  Longitude=0  Date=2023-01-01  Time=10:30:00  GeoTimeZone=-5.0  SunDaylightSaving=off  wind=1  clouds=10  EnableVolumetricClouds=off  CloudCoverage=0  CloudAltitude=6  fog=0  rain=0  RaindropsEffect=off  SnowDensity=0  EnableGeospatial=off  TilesetSource=Earth terrain  UseTrueOrigin=off  OriginHeight=200  OriginLatitude=40.744652  OriginLongitude=-73.988864  MapStyle=Aerial  AdditionalAssetIDs=[]  UseAdvancedSunSky=off  SolarTime=11  TimeZone=-5  Day=21  Month=9  Year=2022  UseDaylightSavingTime=on  DSTStartDay=10  DSTStartMonth=3  DSTEndDay=3  DSTEndMonth=11  DSTSwitchHour=2  sensorTag=MainCamera1  sensorId=1  sensorName=MainCamera1  mountLoc=Origin  offsetFlag=off  tmountOffset=[0, 0, 0]  rmountOffset=[0, 0, 0]  HorizontalResolution=1280  VerticalResolution=720  HorizontalFOV=60  mountPoint=[0 0 0]  mountOrientation=[0 0 0]  aMode=aMode  ID=1  GeoTrigger=Inactive  ViewNameList={'Custom'}  ViewTranslationList={'[0 0 0]'}  ViewRotationList={'[0 0 0]'}
  T Car : Terminator
  T Ground : Terminator
  T LapInfo : Terminator
  T RecCam : Terminator
  T Track : Terminator
  Track : sim3dlib/Simulation 3D Actor  Priority=1  ActorName=Track  ParentName=Scene Origin  Operation=Create at setup  InitScriptText=|  SampleTime=0.05  Translation=[0 0 0]  Rotation=[0 0 0]  Scale=[1 1 1]  aMode=aMode  ActorTag=Track  ActorType=Sim3dActor  ID=2
      | % buildTrackRibbon returns the mesh already in the sim3d LOCAL frame
      | % (y negated, winding reversed), so the actor stays at identity.
      | % 'PlantFrame', true is NOT optional. The Pose block above drives every
      | % actor from VehStateBus x/y/psi, which live in the frame Plant.slx
      | % integrates in; the DEFAULT ribbon is only TRANSLATED onto the racing
      | % line's first point, missing the -psi1 rotation DriverPath applies.
      | % Measured 2026-09-21 against the reference line the car tracks: the
      | % default frame leaves 1048 of 4586 knots off the drawn tarmac at
      | % Barcelona (worst 5.3 m, psi1 = +0.38 deg) and 5001 of 5081 at the
      | % Nurburgring (worst 1032 m, psi1 = -133.03 deg -- the car drives a
      | % kilometre into the grass); with PlantFrame both are 0 of N. Barcelona's
      | % small psi1 is why this survived unnoticed: the first stretch after the
      | % start line registers, and the error only opens up down the lap.
      | rib = buildTrackRibbon('', 'PlantFrame', true);
      | createMesh(Actor, rib.V, rib.N, rib.F, [], rib.C);
      | Actor.TwoSided = true;    % a few quads fold at the hairpin
      | Actor.VertexBlend = 1;    % use the per-vertex kerb/asphalt colours
      | Actor.Shadows = false; Actor.Metallic = 0; Actor.Specular = 0.15;
      | fprintf('Unreal3D/Track: %d vertices, %d faces, %.0f m\n', size(rib.V,1), size(rib.F,1), rib.stats.length);
  Veh Unpack : BusSelector  OutputSignals=x,y,z,psi,roll,pitch,alphaRW_pos,alphaFW_pos,Om_fl,Om_fr,Om_rl,Om_rr
  mode : Constant  Description=Active-choice indicator: 2 = Unreal3D.  Value=2
  spinModeApparent : Constant  Description=vizSpinMode: 1 = apparent wheel spin (cosmetic 30 deg/frame cap, the offline route's default), 0 = physical rate. Display only.
  vizMode : Outport
  wires:
  Ground/1 -> T Ground/1
  Track/1 -> T Track/1
  Car/1 -> T Car/1
  RecCam/1 -> T RecCam/1  "unrealFrame"
  VehState/1 -> Veh Unpack/1
  DriverCmd/1 -> Drv Unpack/1
  LapInfo/1 -> T LapInfo/1
  mode/1 -> vizMode/1
  Veh Unpack/1 -> Pose/1(x)  "<x>"
  Veh Unpack/2 -> Pose/2(y)  "<y>"
  Veh Unpack/3 -> Pose/3(z)  "<z>"
  Veh Unpack/4 -> Pose/4(psi)  "<psi>"
  Veh Unpack/5 -> Pose/5(roll)  "<roll>"
  Veh Unpack/6 -> Pose/6(pitch)  "<pitch>"
  Veh Unpack/7 -> Pose/7(aRWdeg)  "<alphaRW_pos>"
  Veh Unpack/8 -> Pose/8(aFWdeg)  "<alphaFW_pos>"
  Veh Unpack/9 -> Pose/9(OmFL)  "<Om_fl>"
  Veh Unpack/10 -> Pose/10(OmFR)  "<Om_fr>"
  Veh Unpack/11 -> Pose/11(OmRL)  "<Om_rl>"
  Veh Unpack/12 -> Pose/12(OmRR)  "<Om_rr>"
  Drv Unpack/1 -> Pose/13(steer)  "<steer>"
  spinModeApparent/1 -> Pose/14(spinApparent)
  Pose/1(rootT) -> Car/1
  Pose/2(rootR) -> Car/2
  Pose/3(stFL) -> Car/3
  Pose/4(stFR) -> Car/4
  Pose/5(spFL) -> Car/5
  Pose/6(spFR) -> Car/6
  Pose/7(spRL) -> Car/7
  Pose/8(spRR) -> Car/8
  Pose/9(rwR) -> Car/9
  Pose/10(fwHR) -> Car/10
  Pose/11(rwBC) -> Car/11
  Pose/12(fwBCL) -> Car/12
  Pose/13(fwBCR) -> Car/13
  Pose/14(carT) -> CamCarrier/1
  Pose/15(carR) -> CamCarrier/2
  Pose/16(carS) -> CamCarrier/3

== matlab function ARFWr_Sim/Live Instruments/Gear Observer ==
  settings: updateMethod=DISCRETE  sampleTime=0.05
  data: omRL input; gearInd output; omRR input; ratios input; omPk input; omCap input; nHold input
function gearInd = gearObserver(omRL, omRR, ratios, omPk, omCap, nHold)
%#codegen
% DISPLAY-ONLY indicated gear, evaluated live at 0.05 s.
%
% THE CAVEAT THAT MUST TRAVEL WITH THIS NUMBER: Plant.slx models ONE fixed
% effective ratio (vp.gear) and NEVER SHIFTS. The supplier 8-speed table
% pt.gearbox is read by nothing in the plant or the solver. This digit is
% reconstructed from driven-axle wheel speed purely so a viewer has something
% to read, so no shift event, torque interruption, ratio step or inertia
% change exists anywhere in the simulation and NO REPORTED RESULT DEPENDS ON
% IT. Never quote it in a lap-time, shift-strategy or powertrain statement.
%
% Same rule, same parameters and same dwell filter as
% simulink/viz/indicatedGear.m, whose numbers come from the single owner
% indicatedGearParams(pt). ratios/omPk/omCap/nHold arrive as Constant blocks
% reading hudGear fields, so there is no numeric literal in this path.
%
% The rear pair is used because that is the axle the 8-speed physically feeds
% (ICE + P2); the front e-motors sit on a fixed ratio and never see it.

persistent cur cand cnt started

if isempty(started)
    started = false;
    cur     = 1;
    cand    = 1;
    cnt     = 0;
end

n   = numel(ratios);
omW = 0.5*(omRL + omRR);

% candidate crank speeds, masked by the cap -- indicatedGear.m's
% dst(omEng > omCap) = inf
dst    = zeros(1, n);
allOut = true;
for i = 1:n
    omEng = omW * ratios(i);
    if omEng > omCap
        dst(i) = inf;
    else
        dst(i) = abs(omEng - omPk);
        allOut = false;
    end
end

% nearest candidate to omPk. Strict < keeps the FIRST minimum, which is what
% min(dst,[],2) returns offline, including the all-inf case.
raw  = 1;
best = inf;
for i = 1:n
    if dst(i) < best
        best = dst(i);
        raw  = i;
    end
end
if allOut
    raw = n;               % every candidate over the cap -> top gear
end

% First sample seeds the filter with its own raw choice, exactly as the
% offline loop does (cur = raw(1) before the k = 1 iteration).
if ~started
    started = true;
    cur     = raw;
    cand    = raw;
    cnt     = 0;
end

% dwell filter: hold the digit until a new candidate has persisted nHold
% samples. A bare nearest-band rule chatters at every crossover.
if raw == cur
    cnt  = 0;
    cand = cur;
else
    if raw == cand
        cnt = cnt + 1;
    else
        cand = raw;
        cnt  = 1;
    end
    if cnt >= nHold
        cur = cand;
        cnt = 0;
    end
end

gearInd = cur;
end

== matlab function ARFWr_Sim/Visualization/Unreal3D/Pose ==
  settings: updateMethod=DISCRETE  sampleTime=0.05
  data: x input; rootT output; y input; z input; psi input; roll input; pitch input; aRWdeg input; aFWdeg input; OmFL input; OmFR input; OmRL input; OmRR input; steer input; spinApparent input; rootR output; stFL output; stFR output; spFL output; spFR output; spRL output; spRR output; rwR output; fwHR output; rwBC output; fwBCL output; fwBCR output; carT output; carR output; carS output
function [rootT, rootR, stFL, stFR, spFL, spFR, spRL, spRR, rwR, fwHR, rwBC, fwBCL, fwBCR, carT, carR, carS] = Pose(x, y, z, psi, roll, pitch, aRWdeg, aFWdeg, OmFL, OmFR, OmRL, OmRR, steer, spinApparent)
%#codegen
% ISO 8855 body pose in; ISO8855 actor rows out, in metres and DEGREES.
%
% Every actor this feeds is a CHILD of the car root built by
% simulink/viz/zenvoCarActors.m, so each articulation is a LOCAL rotation
% about its own hinge and there is no world-frame plate arithmetic here --
% and therefore no wing anchor literal, in this function or in a Constant
% feeding it. Rotation is DEGREES in every CoordinateSystem mode:
% CoordinateSystem re-maps the AXES, it does not change the unit. Feeding
% radians drew a +15 deg wing at 0.26 deg -- a flat slab -- which is the
% defect this rebuild removes.
%
% The ONE exception is carR, the pose of the invisible camera CARRIER: a
% Simulation 3D Vehicle consumes rotation in radians, so that row and only
% that row is converted.
%
% Wheel spin is integrated here at the block rate and wrapped mod 360.
% spinApparent = 1 applies the COSMETIC cap (30 deg per frame, tanh-shaped)
% that the offline route uses so the rims read as turning instead of
% strobing at 20 Hz. It is never a measurable wheel speed.
%
% The front-flap hinge map has ONE owner, zenvoCarActors('hingeMap'),
% which returns the deploy and tuck end angles. The linear map between them
% is u = (alphaFW + 25)/25, clamped -- the same one line the offline route
% gets as a function handle. The call is extrinsic (simulation only; this
% variant is never code-generated), so the two returns are pre-declared to
% fix their type, CACHED in persistents on the first step, and checked: a
% missing extrinsic would leave the pre-declared zeros behind and silently
% collapse the flap to a dead plate.

coder.extrinsic('zenvoCarActors');
persistent spin dk tk

DT = 0.05;   ZG = 0.02;          % block rate; buildTrackRibbon default ZLift
if isempty(spin), spin = zeros(1,4); end
if isempty(dk) || isempty(tk)
    dk = 0;  tk = 0;
    [dk, tk] = zenvoCarActors('hingeMap');
    % A missing or renamed extrinsic would leave the pre-declared zeros in
    % place, and a hinge map of tuck == deploy == 0 collapses the flap to a
    % dead plate that looks plausible in a render. Fail instead.
    assert(dk ~= tk, 'Pose: zenvoCarActors(''hingeMap'') returned deploy == tuck.');
end

% --- wheel spin -------------------------------------------------------
Om = [OmFL, OmFR, OmRL, OmRR];
if spinApparent > 0.5
    omCap  = deg2rad(30/DT);     % 30 deg per frame, as a rate
    % omHalf is a FIXED constant on this route. The offline route derives it
    % per window (the median |Om| of the window it is playing back); a live
    % causal block has no window to take a median over, so the tanh knee is
    % pinned at 60 rad/s, about 22 m/s on this tyre. The 30 deg/frame cap
    % itself is identical on both routes.
    omHalf = 60;                 % rad/s
    Om = omCap*tanh(Om/omHalf);
end
spin = mod(spin + rad2deg(Om)*DT, 360);

% --- body and wheels --------------------------------------------------
rootT = [x, y, z + ZG];
rootR = rad2deg([roll, pitch, psi]);
sd    = rad2deg(steer);          % DriverCmdBus.steer is the ROAD-WHEEL angle
stFL  = [0, 0, sd];   stFR = [0, 0, sd];
spFL  = [0, spin(1), 0];   spFR = [0, spin(2), 0];
spRL  = [0, spin(3), 0];   spRR = [0, spin(4), 0];

% --- aero surfaces ----------------------------------------------------
% +alpha about the lateral axis lifts the rear plane's trailing edge, i.e.
% a bigger rear-wing angle visibly stands the wing up. rwR drives the PIVOT
% actor (WingRW), whose mesh-carrying child is left alone: the extraction is
% yawed onto ISO first and pitched about the pivot second, and the two do not
% commute. The front flap is hinged at its upper edge, so its station drives
% the HINGE, not the plate, and the two nose strips share that one hinge.
rwR = [0, aRWdeg, 0];
aH  = tk + min(max((aFWdeg + 25)/25, 0), 1)*(dk - tk);
fwHR = [0, aH, 0];

% --- station colours, nearest station to the ACTUAL position ----------
% dashboardApp's palette, so a band can never be drawn in a colour that
% disagrees with the angle its surface is drawn at. The colour goes on the
% BAND actors only -- every surface of this asset is a texture on a white
% material, so painting one would paint over the car's own skin -- and both
% front bands take the same colour because both strips share one hinge.
STA_RW = [-10, 0, 10, 15];
PAL_RW = [0.12 0.47 0.71; 0.50 0.50 0.50; 0.84 0.15 0.16; 1.00 0.60 0.00];
STA_FW = [-25, -20, 0];
PAL_FW = [0.20 0.63 0.79; 0.55 0.55 0.55; 0.55 0.10 0.60];
[~, iR] = min(abs(aRWdeg - STA_RW));
[~, iF] = min(abs(aFWdeg - STA_FW));
rwBC  = PAL_RW(iR, :);
fwBCL = PAL_FW(iF, :);   fwBCR = fwBCL;

% --- invisible camera carrier, engine frame, RADIANS ------------------
carT = zeros(5,3);   carR = zeros(5,3);   carS = 0.001*ones(5,3);
[tE, rE] = isoToSim3d([x, y, z + ZG], [roll, pitch, psi]);   % rE in DEGREES
carT(1,:) = tE;
carR(1,:) = rE*(pi/180);
end
